simulink model "TWIP_model"  (R2019a)
settings: Solver=VariableStepAuto  StartTime=0.0  StopTime=5  RelTol=1e-3
libraries: fuzblock x1, simulink x1
settings Model: Creator=GoodLiar  LastModifiedBy=Duong

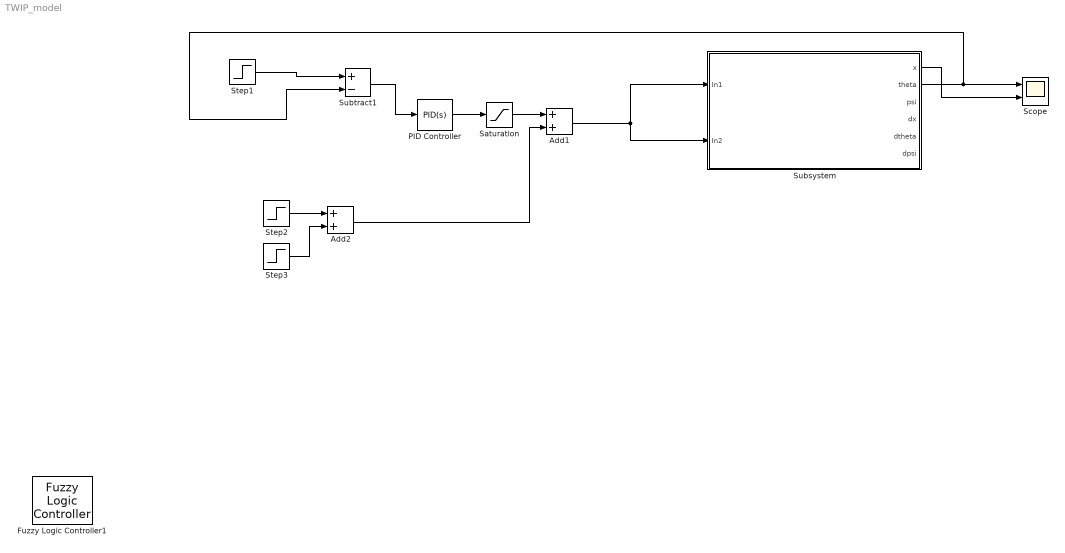
== system TWIP_model ==
  Add1 : Sum
  Add2 : Sum
  Fuzzy Logic Controller1 : fuzblock/Fuzzy Logic  Controller  FIS='1101ver5_sugeno.fis'  OutputSampleNumber=101  DataType=double  FuzzifiedInputs=off  RuleFiringStrengths=off  RuleOutputs=off  AggregatedOutputs=off  SimulateUsing=Interpreted execution  OutOfRangeInputValueMessage=warning  NoRuleFiredMessage=warning  EmptyOutputFuzzySetMessage=warning
  PID Controller : simulink/Continuous/PID Controller  Controller=PID  Form=Parallel  TimeDomain=Continuous-time  SampleTime=-1  IntegratorMethod=Forward Euler  FilterMethod=Forward Euler  ControllerParametersSource=internal  P=-6.26684319828478  I=-9.07996372276762  D=-0.793636829021061  UseFilter=on  N=220.089687018489  TunerSelectOption=Transfer Function Based (PID Tuner App)  InitialConditionSource=internal  InitialConditionForIntegrator=0  InitialConditionForFilter=0  DifferentiatorICPrevScaledInput=0  ExternalReset=none  TrackingMode=off  Kt=1  LimitOutput=off  UpperSaturationLimit=inf  LowerSaturationLimit=-inf  LinearizeAsGain=on  AntiWindupMode=none  Kb=1  POutMin=[]  POutMax=[]  IOutMin=[]  IOutMax=[]  DOutMin=[]  DOutMax=[]  NOutMin=[]  NOutMax=[]  SumOutMin=[]  SumOutMax=[]  SaturationOutMin=[]  SaturationOutMax=[]  PParamMin=[]  PParamMax=[]  IParamMin=[]  IParamMax=[]  DParamMin=[]  DParamMax=[]  NParamMin=[]  NParamMax=[]  KbParamMin=[]  KbParamMax=[]  KtParamMin=[]  KtParamMax=[]  KbOutMin=[]  KbOutMax=[]  KtOutMin=[]  KtOutMax=[]  IntegratorOutMin=[]  IntegratorOutMax=[]  FilterOutMin=[]  FilterOutMax=[]  SumI1OutMin=[]  SumI1OutMax=[]  SumI2OutMin=[]  SumI2OutMax=[]  SumI3OutMin=[]  SumI3OutMax=[]  SumI4OutMin=[]  SumI4OutMax=[]  SumDOutMin=[]  SumDOutMax=[]  DifferentiatorOutMin=[]  DifferentiatorOutMax=[]  FilterDiffOutCoefMin=[]  FilterDiffOutCoefMax=[]  ReciprocalOutMin=[]  ReciprocalOutMax=[]  SumDenOutMin=[]  SumDenOutMax=[]  SumNumOutMin=[]  SumNumOutMax=[]  DivideOutMin=[]  DivideOutMax=[]  IntegratorContinuousStateAttributes=''  IntegratorStateMustResolveToSignalObject=off  IntegratorRTWStateStorageClass=Auto  FilterContinuousStateAttributes=''  FilterStateMustResolveToSignalObject=off  FilterRTWStateStorageClass=Auto  ParallelPVariant=InternalParameters  IdealPVariant=Disabled  IVariant=InternalParameters  DVariant=InternalParameters  IntegratorVariant=Continuous  SatVariant=Disabled  AWVariant=Passthrough  PCopyVariant=Disabled  TRVariant=Disabled  FdbkBlocksVariant=Forward  IdealPFdbkVariant=Disabled  SatFdbkVariant=Disabled  DerivativeFilterVariant=ContFilter  NVariant=InternalParameters  NCopyVariant=Disabled  FilterICVariant=InternalICsFilter  IntegratorICVariant=InternalICs  ExternalResetVariant=Disabled  TRSumVariant=Passthrough  SumFdbkVariant=Disabled  SumVariant=Sum_PID
  Saturation : Saturate  UpperLimit=10  LowerLimit=-10
  Scope : Scope  NumInputPorts=2
  Step1 : Step  After=0  SampleTime=0
  Step2 : Step  Time=10  After=0  SampleTime=0
  Step3 : Step  Time=11  After=0  SampleTime=0
  Subsystem : Subsystem
  Subtract1 : Sum  Inputs=+-
  wires:
  Subsystem/2(theta) -> Subtract1/2, Scope/1
  Step3/1 -> Add2/2
  Step2/1 -> Add2/1
  PID Controller/1 -> Saturation/1
  Step1/1 -> Subtract1/1
  Add2/1 -> Add1/2
  Add1/1 -> Subsystem/2(In2), Subsystem/1(In1)
  Subtract1/1 -> PID Controller/1
  Saturation/1 -> Add1/1
  Subsystem/1("x ") -> Scope/2

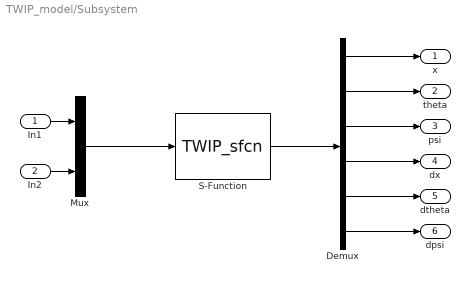
== system TWIP_model/Subsystem ==
  In1 : Inport
  In2 : Inport  Port=2
  Demux : Demux  Outputs=6
  Mux : Mux  Inputs=2
  S-Function : S-Function  FunctionName=TWIP_sfcn  SFunctionDeploymentMode=off  EnableBusSupport=off
  "x " : Outport
  theta : Outport  Port=2
  psi : Outport  Port=3
  dx : Outport  Port=4
  dtheta : Outport  Port=5
  dpsi : Outport  Port=6
  wires:
  Demux/6 -> dpsi/1
  Demux/5 -> dtheta/1
  Mux/1 -> S-Function/1
  Demux/4 -> dx/1
  S-Function/1 -> Demux/1
  Demux/3 -> psi/1
  In1/1 -> Mux/1
  In2/1 -> Mux/2
  Demux/1 -> "x "/1
  Demux/2 -> theta/1
